simulink model "simNRAC"  (R2017b)
settings: Solver=VariableStepAuto  StartTime=0.0  StopTime=100.0  RelTol=1e-3
values from neighbouring files (symbols this model uses):
  D_d = eye(6)*3    [runNRAC.m]
  dragcoeff = [C_d_1, C_d_4, C_d_C, C_d_L, beta, gamma]    [runNRAC.m]
  f_q = [100 50 50 200 100]    [runNRAC.m]
  G_d = eye(6)*0.7    [runNRAC.m]
  k = 0.15    [runNRAC.m]
  M_d = eye(6)*4    [runNRAC.m]
  pos_init = [0 (2*0.77*cos(pi/4)+1) 0]    [runNRAC.m]
  quat_init = eul2quat([0 0 pi],'XYZ')    [runNRAC.m]
  sigma = y_tilde    [plotsNRAC.m]    (also in runNRAC.m = blkdiag(eye(3)*30,eye(3)*30,eye(8)*30))
  theta_init = [0 pi/4 0 pi/4 pi/4 0 pi/4 0]    [runNRAC.m]
  x_init = [pos_init quat_init theta_init zeta_init]'    [runNRAC.m]
undefined symbols (not defined in the file or in its folder): pp, snake
libraries: dspindex x1
settings Model: Creator=sarava  LastModifiedBy=sarava

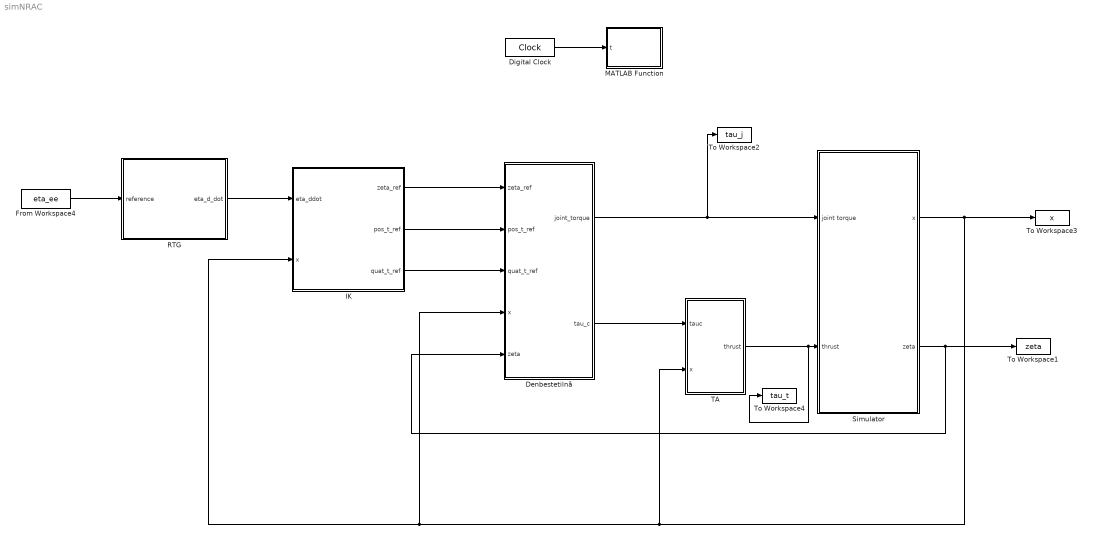
== system simNRAC ==
  Denbestetilnå : Subsystem
  Digital Clock : DigitalClock
  From Workspace4 : FromWorkspace  VariableName=eta_ee  SampleTime=0
  IK : Subsystem
  MATLAB Function : MATLAB Function  TreatAsAtomicUnit=on
  RTG : Subsystem
  Simulator : Subsystem
  TA : Subsystem
  To Workspace1 : ToWorkspace  VariableName=zeta  SaveFormat=Timeseries  SampleTime=-1
  To Workspace2 : ToWorkspace  VariableName=tau_j  SaveFormat=Timeseries  SampleTime=-1
  To Workspace3 : ToWorkspace  VariableName=x  SaveFormat=Timeseries  SampleTime=-1
  To Workspace4 : ToWorkspace  VariableName=tau_t  SaveFormat=Timeseries  SampleTime=-1
  wires:
  RTG/1(eta_d_dot) -> IK/1(eta_ddot)
  TA/1(thrust) -> To Workspace4/1, Simulator/2(thrust)
  Digital Clock/1 -> MATLAB Function/1(t)
  Denbestetilnå/1(joint_torque) -> To Workspace2/1, Simulator/1(joint torque)
  From Workspace4/1 -> RTG/1(reference)
  Denbestetilnå/2("tau_c ") -> TA/1("tauc ")
  IK/1(zeta_ref) -> Denbestetilnå/1(zeta_ref)
  IK/2(pos_t_ref) -> Denbestetilnå/2(pos_t_ref)
  Simulator/1(x) -> Denbestetilnå/4(x), IK/2(x), TA/2("x "), To Workspace3/1
  IK/3(quat_t_ref) -> Denbestetilnå/3(quat_t_ref)
  Simulator/2(zeta) -> Denbestetilnå/5(zeta), To Workspace1/1

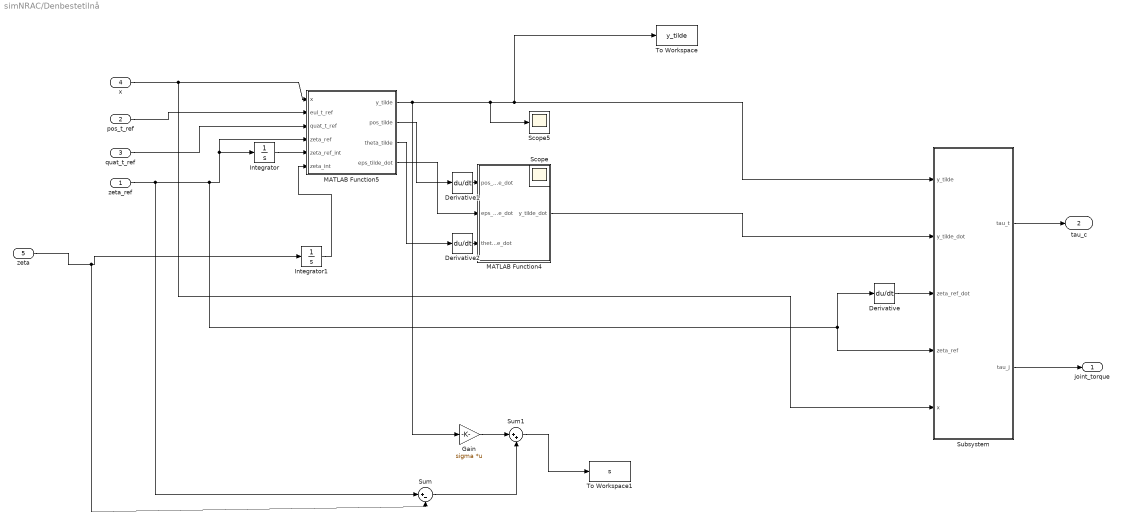
== system simNRAC/Denbestetilnå ==
  zeta_ref : Inport
  pos_t_ref : Inport  Port=2
  quat_t_ref : Inport  Port=3
  x : Inport  Port=4
  zeta : Inport  Port=5
  Derivative : Derivative
  Derivative1 : Derivative
  Derivative2 : Derivative
  Gain : Gain  Gain=sigma  Multiplication=Matrix(K*u) (u vector)
  Integrator : Integrator  InitialCondition=[0 0 0 0 0 0 theta_init]'
  Integrator1 : Integrator  InitialCondition=[0 0 0 0 0 0 theta_init]'
  MATLAB Function4 : MATLAB Function  TreatAsAtomicUnit=on
  MATLAB Function5 : MATLAB Function  TreatAsAtomicUnit=on
  Scope : Scope
  Scope5 : Scope
  Subsystem : Subsystem
  Sum : Sum  Inputs=|+-
  Sum1 : Sum  Inputs=|++
  To Workspace : ToWorkspace  VariableName=y_tilde  SaveFormat=Timeseries  SampleTime=-1
  To Workspace1 : ToWorkspace  VariableName=s  SaveFormat=Timeseries  SampleTime=-1
  joint_torque : Outport
  "tau_c " : Outport  Port=2
  wires:
  quat_t_ref/1 -> MATLAB Function5/3(quat_t_ref)
  pos_t_ref/1 -> MATLAB Function5/2(eul_t_ref)
  zeta_ref/1 -> Sum/1, Derivative/1, Subsystem/4(zeta_ref), MATLAB Function5/4(zeta_ref), Integrator/1
  x/1 -> MATLAB Function5/1(x), Subsystem/5(x)
  Derivative/1 -> Subsystem/3(zeta_ref_dot)
  Integrator/1 -> MATLAB Function5/5(zeta_ref_int)
  zeta/1 -> Integrator1/1, Sum/2
  Subsystem/1(tau_t) -> "tau_c "/1
  Subsystem/2(tau_j) -> joint_torque/1
  Integrator1/1 -> MATLAB Function5/6(zeta_int)
  MATLAB Function5/2(pos_tilde) -> Derivative1/1
  MATLAB Function5/4(eps_tilde_dot) -> MATLAB Function4/2(eps_tilde_dot)
  Derivative2/1 -> MATLAB Function4/3(theta_tilde_dot)
  MATLAB Function5/1(y_tilde) -> Gain/1, Scope5/1, To Workspace/1, Subsystem/1(y_tilde)
  Derivative1/1 -> MATLAB Function4/1(pos_tilde_dot)
  MATLAB Function5/3(theta_tilde) -> Derivative2/1
  MATLAB Function4/1(y_tilde_dot) -> Subsystem/2(y_tilde_dot)
  Sum/1 -> Sum1/2
  Gain/1 -> Sum1/1
  Sum1/1 -> To Workspace1/1

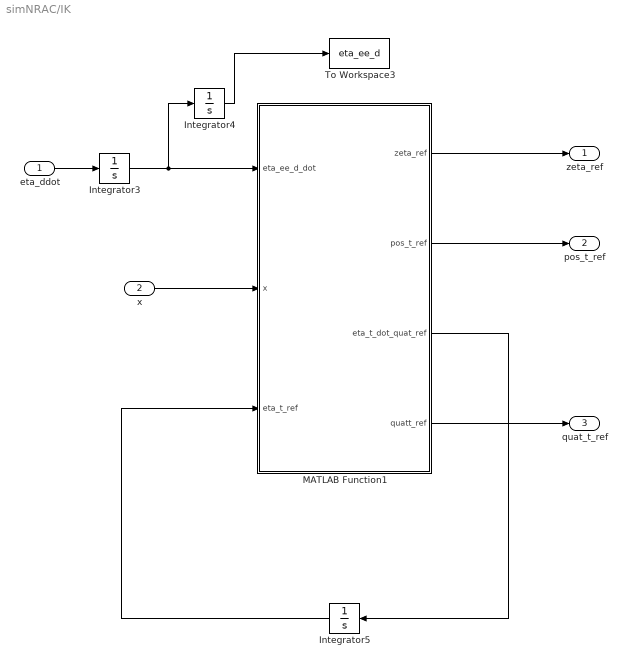
== system simNRAC/IK ==
  eta_ddot : Inport
  x : Inport  Port=2
  Integrator3 : Integrator
  Integrator4 : Integrator
  Integrator5 : Integrator  InitialCondition=[pos_init quat_init]'
  MATLAB Function1 : MATLAB Function  TreatAsAtomicUnit=on
  To Workspace3 : ToWorkspace  VariableName=eta_ee_d  SaveFormat=Timeseries  SampleTime=-1
  zeta_ref : Outport
  pos_t_ref : Outport  Port=2
  quat_t_ref : Outport  Port=3
  wires:
  MATLAB Function1/1(zeta_ref) -> zeta_ref/1
  x/1 -> MATLAB Function1/2(x)
  MATLAB Function1/2(pos_t_ref) -> pos_t_ref/1
  MATLAB Function1/3(eta_t_dot_quat_ref) -> Integrator5/1
  Integrator4/1 -> To Workspace3/1
  Integrator5/1 -> MATLAB Function1/3(eta_t_ref)
  MATLAB Function1/4(quatt_ref) -> quat_t_ref/1
  eta_ddot/1 -> Integrator3/1
  Integrator3/1 -> Integrator4/1, MATLAB Function1/1(eta_ee_d_dot)

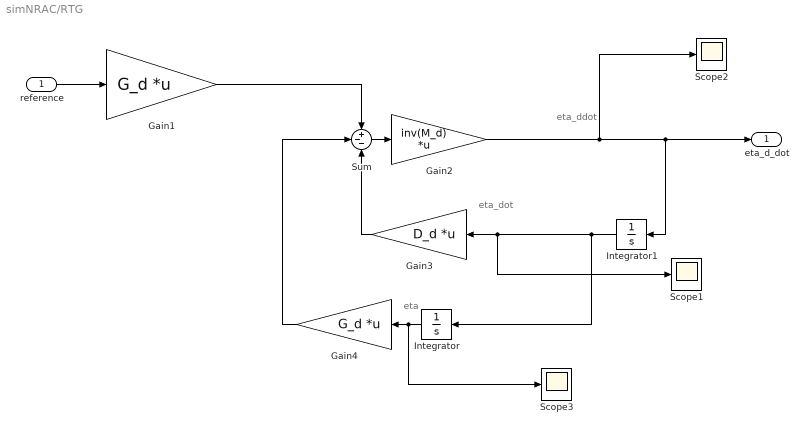
== system simNRAC/RTG ==
  note: eta_dot
  note: eta
  note: eta_ddot
  reference : Inport
  Gain1 : Gain  Gain=G_d  Multiplication=Matrix(K*u) (u vector)
  Gain2 : Gain  Gain=inv(M_d)  Multiplication=Matrix(K*u) (u vector)
  Gain3 : Gain  Gain=D_d  Multiplication=Matrix(K*u) (u vector)
  Gain4 : Gain  Gain=G_d  Multiplication=Matrix(K*u) (u vector)
  Integrator : Integrator
  Integrator1 : Integrator
  Scope1 : Scope
  Scope2 : Scope
  Scope3 : Scope
  Sum : Sum  Inputs=+--
  eta_d_dot : Outport
  wires:
  Gain2/1 -> Scope2/1, eta_d_dot/1, Integrator1/1
  Gain1/1 -> Sum/1
  Sum/1 -> Gain2/1
  reference/1 -> Gain1/1
  Integrator1/1 -> Integrator/1, Scope1/1, Gain3/1
  Integrator/1 -> Scope3/1, Gain4/1
  Gain3/1 -> Sum/3
  Gain4/1 -> Sum/2

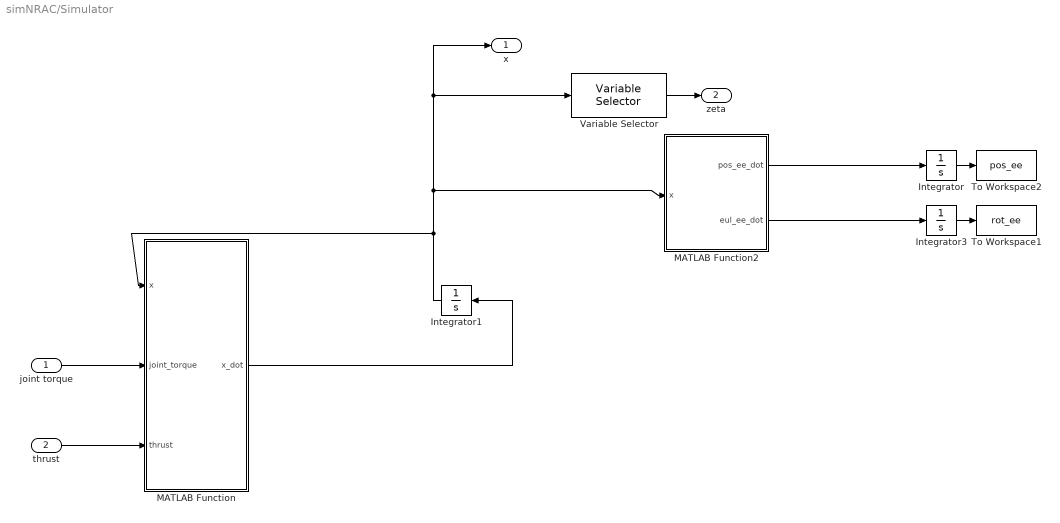
== system simNRAC/Simulator ==
  joint torque : Inport
  thrust : Inport  Port=2
  Integrator : Integrator
  Integrator1 : Integrator  InitialCondition=x_init
  Integrator3 : Integrator
  MATLAB Function : MATLAB Function  TreatAsAtomicUnit=on
  MATLAB Function2 : MATLAB Function  TreatAsAtomicUnit=on
  To Workspace1 : ToWorkspace  VariableName=rot_ee  SaveFormat=Timeseries  SampleTime=-1
  To Workspace2 : ToWorkspace  VariableName=pos_ee  SaveFormat=Timeseries  SampleTime=-1
  Variable Selector : dspindex/Variable Selector  NumInputs=1  rowsOrCols=Rows  IdxMode=Fixed  Elements=16:29  ZerOneIdxMode=One-based  errmode=Clip Index  FillMode=on  FillValues=0
  x : Outport
  zeta : Outport  Port=2
  wires:
  joint torque/1 -> MATLAB Function/2(joint_torque)
  thrust/1 -> MATLAB Function/3(thrust)
  Variable Selector/1 -> zeta/1
  MATLAB Function/1(x_dot) -> Integrator1/1
  Integrator1/1 -> Variable Selector/1, x/1, MATLAB Function2/1(x), MATLAB Function/1(x)
  Integrator/1 -> To Workspace2/1
  MATLAB Function2/1(pos_ee_dot) -> Integrator/1
  MATLAB Function2/2(eul_ee_dot) -> Integrator3/1
  Integrator3/1 -> To Workspace1/1

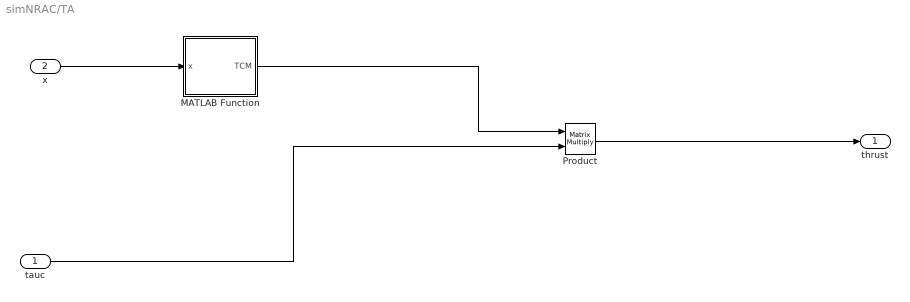
== system simNRAC/TA ==
  "tauc " : Inport
  "x " : Inport  Port=2
  MATLAB Function : MATLAB Function  TreatAsAtomicUnit=on
  Product : Product  Multiplication=Matrix(*)
  thrust : Outport
  wires:
  "x "/1 -> MATLAB Function/1(x)
  MATLAB Function/1(TCM) -> Product/1
  "tauc "/1 -> Product/2
  Product/1 -> thrust/1

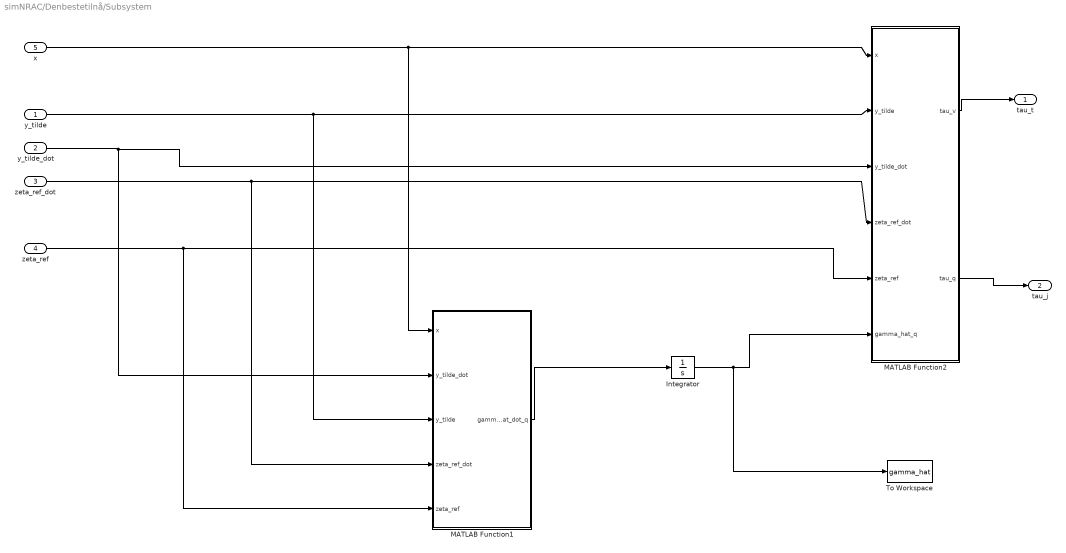
== system simNRAC/Denbestetilnå/Subsystem ==
  y_tilde : Inport
  y_tilde_dot : Inport  Port=2
  zeta_ref_dot : Inport  Port=3
  zeta_ref : Inport  Port=4
  x : Inport  Port=5
  Integrator : Integrator  InitialCondition=[0 0 0 0 0]
  MATLAB Function1 : MATLAB Function  TreatAsAtomicUnit=on
  MATLAB Function2 : MATLAB Function  TreatAsAtomicUnit=on
  To Workspace : ToWorkspace  VariableName=gamma_hat  SaveFormat=Timeseries  SampleTime=-1
  tau_t : Outport
  tau_j : Outport  Port=2
  wires:
  MATLAB Function2/1(tau_v) -> tau_t/1
  MATLAB Function2/2(tau_q) -> tau_j/1
  MATLAB Function1/1(gamma_hat_dot_q) -> Integrator/1
  Integrator/1 -> To Workspace/1, MATLAB Function2/6(gamma_hat_q)
  y_tilde/1 -> MATLAB Function1/3(y_tilde), MATLAB Function2/2(y_tilde)
  zeta_ref/1 -> MATLAB Function2/5(zeta_ref), MATLAB Function1/5(zeta_ref)
  zeta_ref_dot/1 -> MATLAB Function1/4(zeta_ref_dot), MATLAB Function2/4(zeta_ref_dot)
  x/1 -> MATLAB Function1/1(x), MATLAB Function2/1(x)
  y_tilde_dot/1 -> MATLAB Function2/3(y_tilde_dot), MATLAB Function1/2(y_tilde_dot)

== matlab function simNRAC/MATLAB Function ==
  data: t input
function fcn(t)
%#codegen
coder.extrinsic('fprintf');
persistent firstTime

if isempty(firstTime)
    firstTime = false;
    fprintf('Starting Now\n');
end

fprintf('time = %.4f\n',t);

== matlab function simNRAC/Simulator/MATLAB Function ==
  data: x input; x_dot output; joint_torque input; thrust input; pp parameter; snake parameter; dragcoeff parameter
function x_dot  = dyn(x,joint_torque,thrust , pp, snake, dragcoeff)

pos       =  x(1:3);
quat      =  x(4:7);
theta     =  x(8 : 6+snake.n);
zeta      =  x(7+snake.n : 11+2*snake.n);
%Compute rotation matrices and jacobians
[Rcdg,Jcdg]=comp_rot_jac_mcdg(quat,theta,snake);
%Compute mass matrix
M         =  comp_mass(Jcdg,snake);

%Compute relative velocity to take into account the effect of current
velc_h    =  Rcdg(:,:,1)'*pp.velc;
nu        =  zeta(1:6);
zeta(1:3) =  zeta(1:3)-velc_h;

%Compute coriolis, drag, and hydrostatic terms with the relative velocity
[c, d, g] =  comp_cdg(Jcdg,Rcdg,theta,snake,pp,dragcoeff,zeta);
%Compute the thrust-configuration matrix
B         =  comp_TCM(Jcdg,snake);


%Compute the relative acceleration
zeta_dot      =  M\([B [zeros(6,8); eye(8)]]*[thrust;joint_torque]-c-d-g);% -c-d-g

%Remove the effect of current
zeta_dot(1:3) = zeta_dot(1:3)-cross(nu(4:6),velc_h);
%Compute the time derivatives of position and orientation
pos_dot   =  Rcdg(:,:,1)*nu(1:3);  
quat_dot  =  TransAngQ(quat)*nu(4:6)+1*(1-quat'*quat)*quat; 
%Assemble derivative of the state vector
x_dot = [pos_dot ; quat_dot ; zeta(7:snake.n+5) ; zeta_dot];
end

== matlab function simNRAC/TA/MATLAB Function ==
  data: TCM output; x input; snake parameter
function TCM = fcn(x , snake)
quat      =  x(4:7);
theta     =  x(8 : 6+snake.n);
[~, J]    =  comp_rot_jac(quat,theta,snake);
B        =  comp_TCM(J,snake);
TCM_t=B(1:6,:);
TCM=transpose(TCM_t)/(TCM_t*transpose(TCM_t));

== matlab function simNRAC/Simulator/MATLAB Function2 ==
  data: pos_ee_dot output; x input; snake parameter; eul_ee_dot output
function [pos_ee_dot, eul_ee_dot] = snake2points(x,snake)
   quat         = x(4:7);
   theta        = x(8 : 6+snake.n);
    zeta      =  x(7+snake.n : 11+2*snake.n);

   [R,J]=comp_rot_jac(quat,theta,snake);
  
   eul_ee=rotm2eul(R(:,:,10), 'XYZ')';
   Jinv=Jinv_fromeul(eul_ee);
   eta_ee_dot=[R(:,:,10) zeros(3); zeros(3) Jinv]*J(:,:,10)*zeta;
   x_ee_dot=[R(:,:,10) zeros(3); zeros(3) R(:,:,10)]*J(:,:,10)*zeta;
   pos_ee_dot=x_ee_dot(1:3);
   omega_ee=x_ee_dot(4:6);
   eul_ee_dot=eta_ee_dot(4:6);
end

== matlab function simNRAC/Denbestetilnå/MATLAB Function4 ==
  data: pos_tilde_dot input; eps_tilde_dot input; y_tilde_dot output; theta_tilde_dot input
function y_tilde_dot = calc_estdot(pos_tilde_dot,eps_tilde_dot,theta_tilde_dot)

y_tilde_dot=[pos_tilde_dot;eps_tilde_dot;theta_tilde_dot];
end

== matlab function simNRAC/Denbestetilnå/Subsystem/MATLAB Function1 ==
  data: x input; y_tilde_dot input; y_tilde input; zeta_ref_dot input; zeta_ref input; gamma_hat_dot_q output; sigma parameter; k parameter; f_q parameter; snake parameter
function gamma_hat_dot_q  = input(x, y_tilde_dot, y_tilde,zeta_ref_dot, zeta_ref,sigma, k, f_q,snake)


quat      =  x(4:7);
gamma_hat_dot_v=zeros(5,1);
gamma_hat_dot_q=zeros(5,1);
zeta      =  x(7+snake.n : 11+2*snake.n);
zeta_tilde=zeta_ref-zeta;


phi=[zeta_ref_dot zeta ones(14,1)*k y_tilde_dot y_tilde];


s_q=zeta_tilde+sigma*y_tilde;


for i=1:5
gamma_hat_dot_q(i)=f_q(i)*norm(s_q)*norm(phi(:,i));
end

== matlab function simNRAC/IK/MATLAB Function1 ==
  data: eta_ee_d_dot input; x input; eta_t_ref input; zeta_ref output; snake parameter; pos_t_ref output; eta_t_dot_quat_ref output; quatt_ref output
function [zeta_ref , pos_t_ref,eta_t_dot_quat_ref, quatt_ref] = fucn(eta_ee_d_dot,x,eta_t_ref, snake)
quat      =  x(4:7);
theta     =  x(8 : 6+snake.n);
[R, J_t]    =  comp_rot_jac(quat,theta,snake);


eul_ee=rotm2eul(R(:,:,10), 'XYZ')';

Jinv=Jinv_fromeul(eul_ee);
J=[R(:,:,10) zeros(3); zeros(3) Jinv]*J_t(:,:,10);

zeta_ref=J'/(J*J'+0.0001*eye(6))*(eta_ee_d_dot);%+K*sigma_tilde);
eta_ee_ref_dot=J*zeta_ref;



quatt_ref=eta_t_ref(4:7);
pos_t_ref=eta_t_ref(1:3);
R_tail=quat2rotm(quatt_ref');

pos_t_dot   =  R_tail(:,:,1)*zeta_ref(1:3);  
quat_t_dot  =  TransAngQ(quatt_ref)*zeta_ref(4:6)+1*(1-quatt_ref'*quatt_ref)*quatt_ref; 

eta_t_dot_quat_ref=[pos_t_dot; quat_t_dot];
end

== matlab function simNRAC/Denbestetilnå/Subsystem/MATLAB Function2 ==
  data: x input; y_tilde input; y_tilde_dot input; zeta_ref_dot input; zeta_ref input; gamma_hat_q input; tau_v output; tau_q output; sigma parameter; k parameter; snake parameter
function [tau_v,tau_q]= input(x, y_tilde,y_tilde_dot, zeta_ref_dot,zeta_ref, gamma_hat_q, sigma, k,snake)


tau=zeros(14,1);
tauv=zeros(5,1);





out=zeros(14,1);


quat      =  x(4:7);

zeta      =  x(7+snake.n : 11+2*snake.n);
zeta_tilde=zeta_ref-zeta;


phi=[zeta_ref_dot zeta ones(14,1)*k y_tilde_dot y_tilde];

s_q=zeta_tilde+sigma*y_tilde;

for j=1:5
    norms=norm(s_q);
    normphi=norm(phi(:,j));     
    if norms<0.01
        norms=0.01;
    end
     if normphi<0.01
        normphi=0.01;
     end
    normq=norms*normphi;
    if j==5
        K_q=gamma_hat_q(j)*s_q*phi(:,j)'/(normq);
        tau=tau+K_q*phi(:,j);
    else
        K_q=gamma_hat_q(j)*s_q*phi(:,j)'/(normq);
        tau=tau+K_q*phi(:,j);
    end
end




% 

 theta=x(8:15);
 [R, J]    =  comp_rot_jac(quat,theta,snake);
 B=comp_TCM(J,snake);
 B_u=[eye(6,6) zeros(6,8); B(7:end,:)*pinv(B(1:6,:)) eye(8)];
 
u=pinv(B_u)*tau;%
tau_v=u(1:6);
tau_q=u(7:14);

== matlab function simNRAC/Denbestetilnå/MATLAB Function5 ==
  data: x input; y_tilde output; eul_t_ref input; quat_t_ref input size=4; zeta_ref input; zeta_ref_int input; snake parameter; zeta_int input; pos_tilde output; theta_tilde output; eps_tilde_dot output
function [y_tilde,pos_tilde,theta_tilde,eps_tilde_dot]  = dyn(x,eul_t_ref, quat_t_ref, zeta_ref,zeta_ref_int,snake, zeta_int)
pos_t       =  x(1:3);
quat      =  x(4:7);
theta     =  x(8 : 6+snake.n);
zeta      =  x(7+snake.n : 11+2*snake.n);

pos_t_ref=eul_t_ref(1:3);
pos_tilde=RotQ(quat)*(pos_t_ref-pos_t);%
pos_tilde2=quat2rotm(quat')*(pos_t_ref-pos_t);


quat_tilde=quat(1)*quat_t_ref(2:4)-quat_t_ref(1)*quat(2:4)+cross(quat_t_ref(2:4),quat(2:4));
eta_tilde = quat(1) * quat_t_ref (1) + quat_t_ref(2:4)'*quat(2:4);
if eta_tilde < 0
quat_tilde = - quat_tilde ;
end

theta_tilde=zeta_ref_int(7:14)-zeta_int(7:14);


y_tilde=[pos_tilde;quat_tilde;theta_tilde];


nu2_tilde=zeta_ref(4:6)-zeta(4:6);
eps_tilde_dot=0.5*eta_tilde*nu2_tilde + 0.5*skew(quat_tilde)*nu2_tilde;

end
